simulink model "NOx_SCR_Guidline_Model"  (R2019a)
settings: Solver=FixedStepDiscrete  StartTime=0.0  StopTime=10.0  FixedStep=0.1  RelTol=1e-3
undefined symbols (not defined in the file or in its folder): Actual_Injector_on, Flow_rate_min, Injector_off, injector_On_counter, Req_Downstrem_nox, Req_ON, Req_SCR_Bed_temp, Required_injector_On, Required_pressure
settings Model: Creator=Kore  LastModifiedBy=Kore
settings OptimizationCC: DefaultParameterBehavior=Inlined  UseDivisionForNetSlopeComputation=on  EnhancedBackFolding=on  PassReuseOutputArgsAs=Individual arguments  OptimizeBlockOrder=speed  DifferentSizesBufferReuse=on  OptimizationCustomize=off
settings DebuggingCC: SignalInfNanChecking=error  ParameterTunabilityLossMsg=error  UniqueDataStoreMsg=warning  AssertControl=DisableAll  StrictBusMsg=ErrorOnBusTreatedAsVector  SFUndirectedBroadcastEventsDiag=error
settings SFSimCC: CompileTimeRecursionLimit=0  EnableRuntimeRecursion=off  MATLABDynamicMemAlloc=off
settings RTWCC: SystemTargetFile=ert.tlc  TemplateMakefile=ert_default_tmf  GenerateReport=on  IncludeHyperlinkInReport=on  LaunchReport=on  GenerateTraceInfo=on  GenerateTraceReport=on  GenerateTraceReportSl=on  GenerateTraceReportSf=on  GenerateTraceReportEml=on
settings CodeAppCC: ForceParamTrailComments=on  IgnoreCustomStorageClasses=off  OperatorAnnotations=on  SimulinkDataObjDesc=on  SFDataObjDesc=on  MATLABFcnDesc=on  InsertBlockDesc=on
settings ERTTargetCC: TargetLangStandard=C99 (ISO)  UtilityFuncGeneration=Shared location  GenerateSampleERTMain=on  SupportNonFinite=off  ParenthesesLevel=Maximum  CastingMode=Standards  GenerateSharedConstants=off  InlinedParameterPlacement=NonHierarchical  ERTCustomFileTemplate=example_file_process.tlc  EnableSignedLeftShifts=off  EnableSignedRightShifts=off
settings ConfigComp: DVMode=DesignErrorDetection  DVMaxProcessTime=900  DVTestSuiteOptimization=Auto  DVDetectDeadLogic=on  DVDetectActiveLogic=on  DVDetectOutOfBounds=on  DVRebuildModelRepresentation=Always

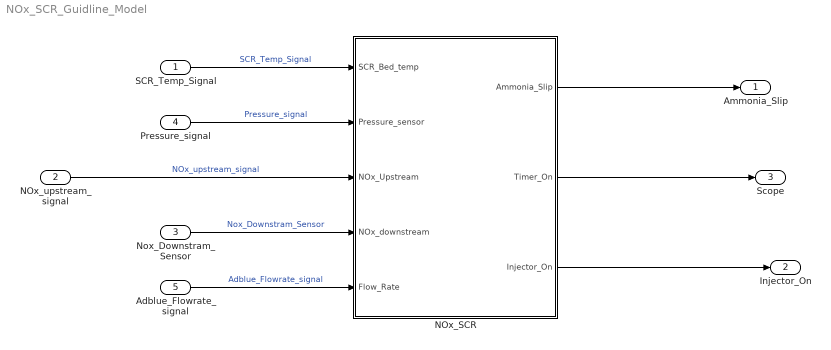
== system NOx_SCR_Guidline_Model ==
  SCR_Temp_Signal : Inport
  NOx_upstream_signal : Inport  Port=2
  Nox_Downstram_Sensor : Inport  Port=3
  Pressure_signal : Inport  Port=4
  Adblue_Flowrate_signal : Inport  Port=5
  NOx_SCR : Subsystem
  Ammonia_Slip : Outport
  Injector_On : Outport  Port=2
  Scope : Outport  Port=3
  wires:
  SCR_Temp_Signal/1 -> NOx_SCR/1(SCR_Bed_temp)  "SCR_Temp_Signal"
  NOx_SCR/3(Injector_On) -> Injector_On/1
  Nox_Downstram_Sensor/1 -> NOx_SCR/4(NOx_downstream)  "Nox_Downstram_Sensor"
  Pressure_signal/1 -> NOx_SCR/2(Pressure_sensor)  "Pressure_signal"
  NOx_SCR/2(Timer_On) -> Scope/1
  NOx_SCR/1(Ammonia_Slip) -> Ammonia_Slip/1
  Adblue_Flowrate_signal/1 -> NOx_SCR/5(Flow_Rate)  "Adblue_Flowrate_signal"
  NOx_upstream_signal/1 -> NOx_SCR/3(NOx_Upstream)  "NOx_upstream_signal"

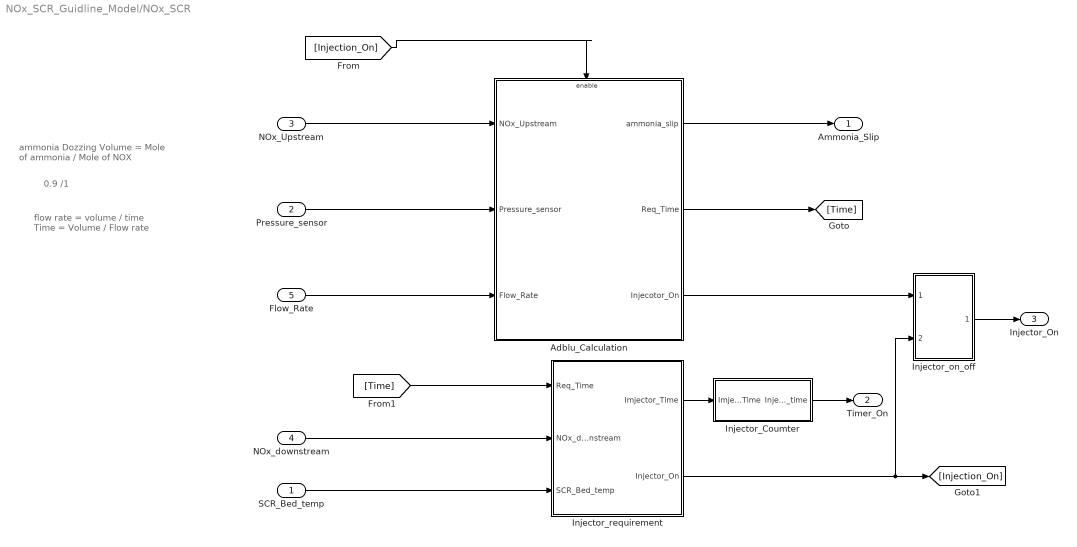
== system NOx_SCR_Guidline_Model/NOx_SCR ==
  note: 0.9 /1
  note: ammonia Dozzing Volume =
      |  Mole of ammonia / Mole of NOX
  note: flow rate = volume / time
      |
      | Time = Volume / Flow rate
  SCR_Bed_temp : Inport
  Pressure_sensor : Inport  Port=2
  NOx_Upstream : Inport  Port=3
  NOx_downstream : Inport  Port=4
  Flow_Rate : Inport  Port=5
  Adblu_Calculation : Subsystem
  Injector_Coumter : Subsystem
  Injector_on_off : Subsystem
  Injector_requirement : Subsystem
  Ammonia_Slip : Outport
  Timer_On : Outport  Port=2
  Injector_On : Outport  Port=3
  wires:
  NOx_Upstream/1 -> Adblu_Calculation/1(NOx_Upstream)
  Pressure_sensor/1 -> Adblu_Calculation/2(Pressure_sensor)
  Adblu_Calculation/1(ammonia_slip) -> Ammonia_Slip/1
  NOx_downstream/1 -> Injector_requirement/2(NOx_downstream)
  [Injection_On] -> Adblu_Calculation/Enable
  Injector_Coumter/1(Injector_injection_time) -> Timer_On/1
  SCR_Bed_temp/1 -> Injector_requirement/3(SCR_Bed_temp)
  Injector_requirement/1(Imjector_Time) -> Injector_Coumter/1(Imjector_Time)
  Adblu_Calculation/2(Req_Time) -> [Time]
  [Time] -> Injector_requirement/1(Req_Time)
  Injector_requirement/2(Injector_On) -> Injector_on_off/2(Condition_Of_Injector), [Injection_On]
  Flow_Rate/1 -> Adblu_Calculation/3(Flow_Rate)
  Adblu_Calculation/3(Injecotor_On) -> Injector_on_off/1(injector_On)
  Injector_on_off/1(On_injector) -> Injector_On/1

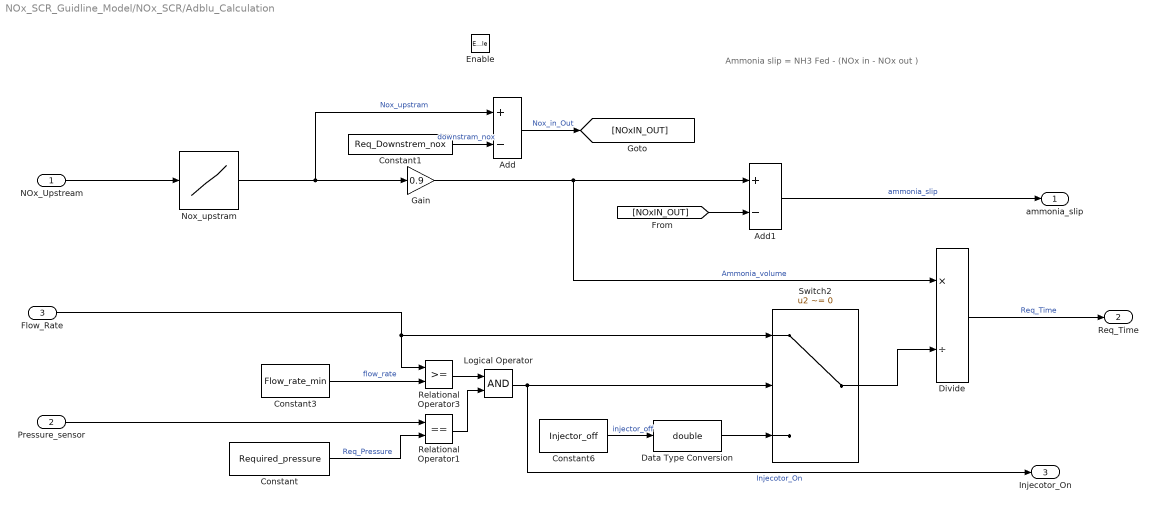
== system NOx_SCR_Guidline_Model/NOx_SCR/Adblu_Calculation ==
  note: Ammonia slip = NH3 Fed - (NOx in - NOx out )
  NOx_Upstream : Inport
  Pressure_sensor : Inport  Port=2
  Flow_Rate : Inport  Port=3
  Enable : EnablePort  StatesWhenEnabling=reset
  Add : Sum  Inputs=+-
  Add1 : Sum  Inputs=+-
  Constant : Constant  Value=Required_pressure
  Constant1 : Constant  Value=Req_Downstrem_nox
  Constant3 : Constant  Value=Flow_rate_min
  Constant6 : Constant  Value=Injector_off
  Data Type Conversion : DataTypeConversion  OutDataTypeStr=double
  Divide : Product  Inputs=*/  OutDataTypeStr=double  RndMeth=Round
  Gain : Gain  Gain=0.9
  Logical Operator : Logic  AllPortsSameDT=off  OutDataTypeStr=boolean
  Nox_upstram : Lookup_n-D  NumberOfTableDimensions=1  BreakpointsForDimension1=|  BreakpointsForDimension1DataTypeStr=double  Table=|  TableDataTypeStr=double  IntermediateResultsDataTypeStr=double  InternalRulePriority=Speed  OutDataTypeStr=double  InputSameDT=on
      BreakpointsForDimension1=|
      | [10
      | 70
      | 77.6
      | 80.4
      | 86.4
      | 99.6
      | 108
      | 117.6
      | 127.2
      | 136.8
      | 149.3
      | 158.3
      | 163.3
      | 168.3
      | 175.3
      | 181.5
      | 187.7
      | 193.9
      | 200.1
      | 206.3
      | 212.85
      | 223.5
      | 233.15
      | 242.8
      | 255.45
      | 264.9
      | 275.35
      | 285.8
      | 296.25
      | 306.7
      | 317.15
      | 327.6
      | 338.05
      | 348.5
      | 358.95
      | 369.4
      | 379.85
      | 390.3
      | 400.75
      | 411.2
      | 421.65
      | 432.1
      | 442.55
      | 453
      | 463.45
      | 473.9
      | 484.35
      | 494.8
      | 505.25
      | 515.7
      | 526.15
      | 536.6
      | 547.05
      | 557.5
      | 567.95
      | 578.4
      | 588.85
      | 599.3
      | 609.75
      | 620.2
      | 630.65
      | 641.1
      | 651.55
      | 662
      | 672.45
      | 682.9
      | 693.35
      | 703.8
      | ]
      Table=|
      | [10
      | 70
      | 77.6
      | 80.4
      | 86.4
      | 99.6
      | 108
      | 117.6
      | 127.2
      | 136.8
      | 149.3
      | 158.3
      | 163.3
      | 168.3
      | 175.3
      | 181.5
      | 187.7
      | 193.9
      | 200.1
      | 206.3
      | 212.85
      | 223.5
      | 233.15
      | 242.8
      | 255.45
      | 264.9
      | 275.35
      | 285.8
      | 296.25
      | 306.7
      | 317.15
      | 327.6
      | 338.05
      | 348.5
      | 358.95
      | 369.4
      | 379.85
      | 390.3
      | 400.75
      | 411.2
      | 421.65
      | 432.1
      | 442.55
      | 453
      | 463.45
      | 473.9
      | 484.35
      | 494.8
      | 505.25
      | 515.7
      | 526.15
      | 536.6
      | 547.05
      | 557.5
      | 567.95
      | 578.4
      | 588.85
      | 599.3
      | 609.75
      | 620.2
      | 630.65
      | 641.1
      | 651.55
      | 662
      | 672.45
      | 682.9
      | 693.35
      | 703.8
      | ]
  Relational Operator1 : RelationalOperator  Operator===  RndMeth=Simplest
  Relational Operator3 : RelationalOperator  OutDataTypeStr=boolean  RndMeth=Simplest
  Switch2 : Switch  Criteria=u2 ~= 0
  ammonia_slip : Outport
  Req_Time : Outport  Port=2
  Injecotor_On : Outport  Port=3
  wires:
  Pressure_sensor/1 -> Relational Operator1/1
  Relational Operator1/1 -> Logical Operator/2
  Constant/1 -> Relational Operator1/2  "Req_Pressure"
  NOx_Upstream/1 -> Nox_upstram/1
  Constant3/1 -> Relational Operator3/2  "flow_rate"
  Relational Operator3/1 -> Logical Operator/1
  Constant6/1 -> Data Type Conversion/1  "injector_off"
  Logical Operator/1 -> Injecotor_On/1, Switch2/2  "Injecotor_On"
  [NOxIN_OUT] -> Add1/2
  Flow_Rate/1 -> Relational Operator3/1, Switch2/1
  Add1/1 -> ammonia_slip/1  "ammonia_slip"
  Gain/1 -> Divide/1, Add1/1  "Ammonia_volume"
  Nox_upstram/1 -> Gain/1, Add/1  "Nox_upstram"
  Add/1 -> [NOxIN_OUT]  "Nox_in_Out"
  Constant1/1 -> Add/2  "downstram_nox"
  Switch2/1 -> Divide/2
  Divide/1 -> Req_Time/1  "Req_Time"
  Data Type Conversion/1 -> Switch2/3

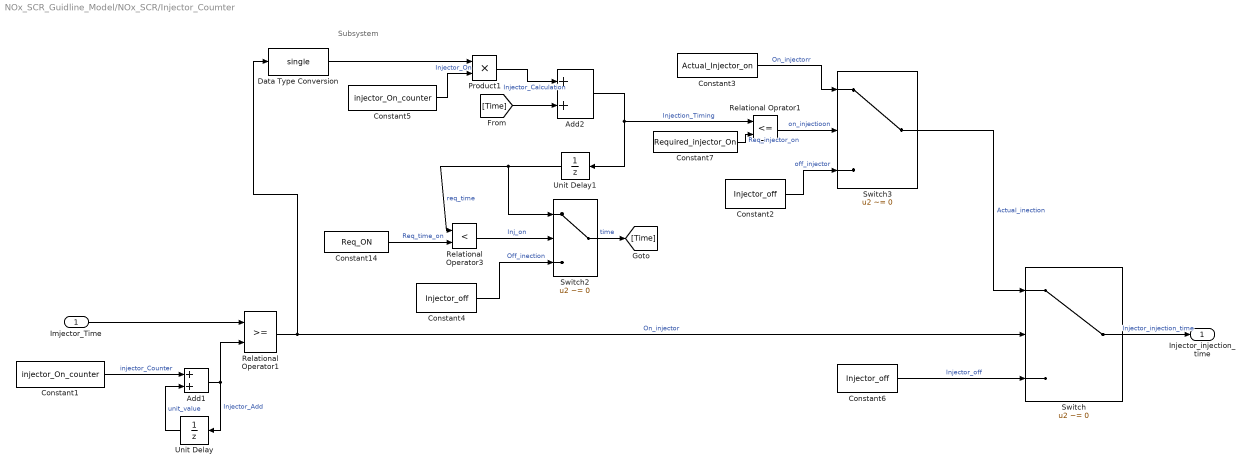
== system NOx_SCR_Guidline_Model/NOx_SCR/Injector_Coumter ==
  note: Subsystem
  Imjector_Time : Inport
  Add1 : Sum
  Add2 : Sum
  Constant1 : Constant  Value=injector_On_counter
  Constant14 : Constant  Value=Req_ON
  Constant2 : Constant  Value=Injector_off
  Constant3 : Constant  Value=Actual_Injector_on
  Constant4 : Constant  Value=Injector_off
  Constant5 : Constant  Value=injector_On_counter
  Constant6 : Constant  Value=Injector_off
  Constant7 : Constant  Value=Required_injector_On
  Data Type Conversion : DataTypeConversion  OutDataTypeStr=single
  Product1 : Product
  Relational Operator1 : RelationalOperator  OutDataTypeStr=boolean  RndMeth=Simplest
  Relational Operator3 : RelationalOperator  Operator=<  OutDataTypeStr=boolean  RndMeth=Simplest
  Relational Oprator1 : RelationalOperator  Operator=<=  OutDataTypeStr=boolean  RndMeth=Simplest
  Switch : Switch  Criteria=u2 ~= 0
  Switch2 : Switch  Criteria=u2 ~= 0
  Switch3 : Switch  Criteria=u2 ~= 0
  Unit Delay : UnitDelay  SampleTime=-1  HasFrameUpgradeWarning=on
  Unit Delay1 : UnitDelay  SampleTime=-1  HasFrameUpgradeWarning=on
  Injector_injection_time : Outport
  wires:
  Constant6/1 -> Switch/3  "Injector_off"
  Unit Delay/1 -> Add1/2  "unit_value"
  Constant1/1 -> Add1/1  "injector_Counter"
  Add1/1 -> Unit Delay/1, Relational Operator1/2  "Injector_Add"
  Switch3/1 -> Switch/1  "Actual_inection"
  Switch/1 -> Injector_injection_time/1  "Injector_injection_time"
  Add2/1 -> Relational Oprator1/1, Unit Delay1/1  "Injection_Timing"
  Relational Oprator1/1 -> Switch3/2  "on_injectioon"
  [Time] -> Add2/2
  Constant2/1 -> Switch3/3  "off_injector"
  Relational Operator1/1 -> Data Type Conversion/1, Switch/2  "On_injector"
  Constant4/1 -> Switch2/3  "Off_inection"
  Constant14/1 -> Relational Operator3/2  "Req_time_on"
  Product1/1 -> Add2/1  "Injector_Calculation"
  Switch2/1 -> [Time]  "time"
  Constant5/1 -> Product1/2  "Injector_On"
  Constant7/1 -> Relational Oprator1/2  "Req_injector_on"
  Constant3/1 -> Switch3/1  "On_injectorr"
  Relational Operator3/1 -> Switch2/2  "Inj_on"
  Unit Delay1/1 -> Relational Operator3/1, Switch2/1  "req_time"
  Data Type Conversion/1 -> Product1/1
  Imjector_Time/1 -> Relational Operator1/1

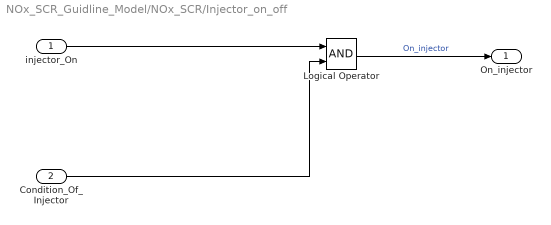
== system NOx_SCR_Guidline_Model/NOx_SCR/Injector_on_off ==
  injector_On : Inport
  Condition_Of_Injector : Inport  Port=2
  Logical Operator : Logic  AllPortsSameDT=off  OutDataTypeStr=boolean
  On_injector : Outport
  wires:
  Logical Operator/1 -> On_injector/1  "On_injector"
  Condition_Of_Injector/1 -> Logical Operator/2
  injector_On/1 -> Logical Operator/1

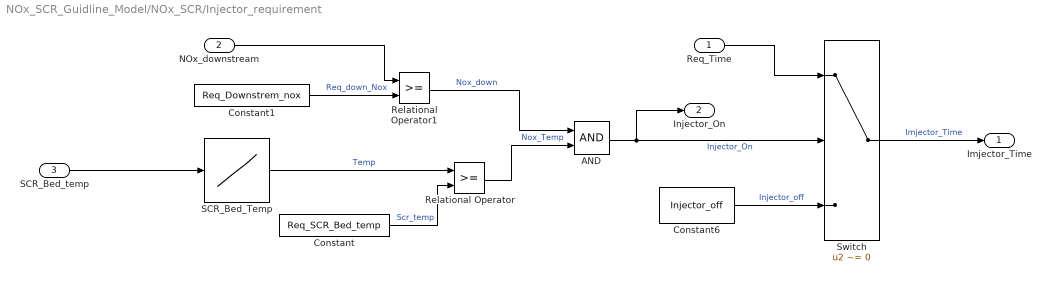
== system NOx_SCR_Guidline_Model/NOx_SCR/Injector_requirement ==
  Req_Time : Inport
  NOx_downstream : Inport  Port=2
  SCR_Bed_temp : Inport  Port=3
  AND : Logic  AllPortsSameDT=off  OutDataTypeStr=boolean
  Constant : Constant  Value=Req_SCR_Bed_temp
  Constant1 : Constant  Value=Req_Downstrem_nox
  Constant6 : Constant  Value=Injector_off
  Relational Operator : RelationalOperator  OutDataTypeStr=boolean  RndMeth=Simplest
  Relational Operator1 : RelationalOperator  OutDataTypeStr=boolean  RndMeth=Simplest
  SCR_Bed_Temp : Lookup_n-D  NumberOfTableDimensions=1  BreakpointsForDimension1=[1:10:650]  BreakpointsForDimension2=[1:1:500]  BreakpointsForDimension1DataTypeStr=double  Table=[1:10:650]  TableDataTypeStr=double  IntermediateResultsDataTypeStr=double  InternalRulePriority=Speed  OutDataTypeStr=double  InputSameDT=on
  Switch : Switch  Criteria=u2 ~= 0
  Imjector_Time : Outport
  Injector_On : Outport  Port=2
  wires:
  Constant1/1 -> Relational Operator1/2  "Req_down_Nox"
  Constant/1 -> Relational Operator/2  "Scr_temp"
  Constant6/1 -> Switch/3  "Injector_off"
  SCR_Bed_Temp/1 -> Relational Operator/1  "Temp"
  AND/1 -> Injector_On/1, Switch/2  "Injector_On"
  Relational Operator1/1 -> AND/1  "Nox_down"
  Relational Operator/1 -> AND/2  "Nox_Temp"
  SCR_Bed_temp/1 -> SCR_Bed_Temp/1
  Switch/1 -> Imjector_Time/1  "Imjector_Time"
  NOx_downstream/1 -> Relational Operator1/1
  Req_Time/1 -> Switch/1
